simulink model "SkywalkerX8_Longitudinal_Control_Digital"  (R2018a)
settings: Solver=FixedStepAuto  StartTime=0.0  StopTime=inf  FixedStep=0.001  RelTol=1e-3
undefined symbols (not defined in the file): DiscIntNeverNeededParam, SkywalkerX8
libraries: simulink_extras x4
settings Model: EnablePacing=on  Creator=David  LastModifiedBy=David

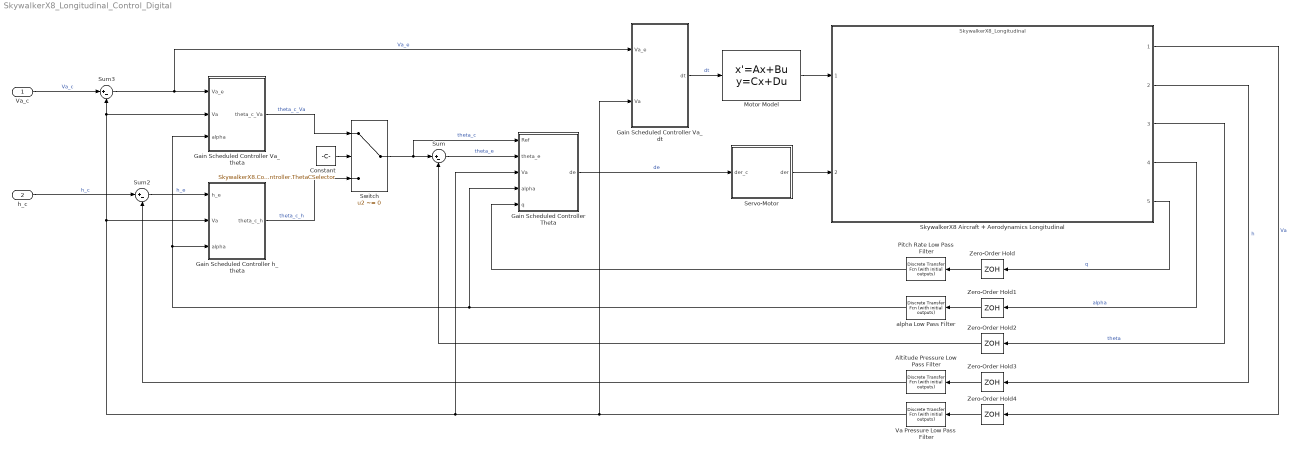
== system SkywalkerX8_Longitudinal_Control_Digital ==
  Va_c : Inport
  h_c : Inport  Port=2
  Altitude Pressure Low Pass Filter : simulink_extras/Additional Discrete/Discrete Transfer Fcn (with initial outputs)  N=cell2mat(SkywalkerX8.Sensors.Filters.AltitudePressure.FilterTFDigital.Numerator)  D=cell2mat(SkywalkerX8.Sensors.Filters.AltitudePressure.FilterTFDigital.Denominator)  U0=-SkywalkerX8.InitialConditions.XeYeZe(3)  Y0=-SkywalkerX8.InitialConditions.XeYeZe(3)  TS=SkywalkerX8.Sensors.Filters.AltitudePressure.FilterSampleTime
      settings: SourceProductName=Simulink  SourceProductBaseCode=SL
  Constant : Constant  Value=SkywalkerX8.Control.Longitudinal.AlgebraicDesign.ReducedOrderModel.Controller.ThetaCSelector
  Gain Scheduled Controller Theta : Subsystem
  Gain Scheduled Controller Va_dt : Subsystem
  Gain Scheduled Controller Va_theta : Subsystem
  Gain Scheduled Controller h_theta : Subsystem
  Motor Model : StateSpace  A=SkywalkerX8.Actuators.Motor.SS.A  B=SkywalkerX8.Actuators.Motor.SS.B  C=SkywalkerX8.Actuators.Motor.SS.C  D=SkywalkerX8.Actuators.Motor.SS.D  InitialCondition=SkywalkerX8.InitialConditions.dt/SkywalkerX8.Actuators.Motor.SS.C
      mask Display: image('motor.jpg', 'center')
  Pitch Rate Low Pass Filter : simulink_extras/Additional Discrete/Discrete Transfer Fcn (with initial outputs)  N=cell2mat(SkywalkerX8.Sensors.Filters.AngularRates.Pitch.FilterTFDigital.Numerator)  D=cell2mat(SkywalkerX8.Sensors.Filters.AngularRates.Pitch.FilterTFDigital.Denominator)  U0=SkywalkerX8.Sensors.Filters.AngularRates.Pitch.InitialCondition  Y0=SkywalkerX8.Sensors.Filters.AngularRates.Pitch.InitialCondition  TS=SkywalkerX8.Sensors.Filters.AngularRates.Pitch.FilterSampleTime
      settings: SourceProductName=Simulink  SourceProductBaseCode=SL
  Servo-Motor : Subsystem
      mask Display: image('servo.jpg', 'center')
  SkywalkerX8 Aircraft + Aerodynamics Longitudinal : ModelReference  ModelNameDialog=SkywalkerX8_Longitudinal  ModelReferenceVersion=1.60
      mask Display:
      | image('x8SkySunset.png', 'center')
      | 
      | port_label('input', 1, '\delta_t (Unitless)', 'texmode', 'on')
      | port_label('input', 2, '\delta_e (rad)', 'texmode', 'on')
      | 
      | port_label('output', 1, 'V_a (m/s)', 'texmode', 'on')
      | port_label('output', 2, 'Altitude (m)', 'texmode', 'on')
      | port_label('output', 3, '\theta (rad)', 'texmode', 'on')
      | port_label('output', 4, 'alpha (rad)', 'texmode', 'on')
      | port_label('output', 5, 'q (rad/s)', 'texmode', 'on')
  Sum : Sum  Inputs=|+-
  Sum2 : Sum  Inputs=|+-
  Sum3 : Sum  Inputs=|+-
  Switch : Switch  Criteria=u2 ~= 0
  Va Pressure Low Pass Filter : simulink_extras/Additional Discrete/Discrete Transfer Fcn (with initial outputs)  N=cell2mat(SkywalkerX8.Sensors.Filters.AirspeedPressure.FilterTFDigital.Numerator)  D=cell2mat(SkywalkerX8.Sensors.Filters.AirspeedPressure.FilterTFDigital.Denominator)  U0=sqrt(SkywalkerX8.InitialConditions.uvw*SkywalkerX8.InitialConditions.uvw')  Y0=sqrt(SkywalkerX8.InitialConditions.uvw*SkywalkerX8.InitialConditions.uvw')  TS=SkywalkerX8.Sensors.Filters.AirspeedPressure.FilterSampleTime
      settings: SourceProductName=Simulink  SourceProductBaseCode=SL
  Zero-Order Hold : ZeroOrderHold  SampleTime=SkywalkerX8.Sensors.IMU.Gyroscope.SampleTime
  Zero-Order Hold1 : ZeroOrderHold  SampleTime=SkywalkerX8.Sensors.AoA.SampleTime
  Zero-Order Hold2 : ZeroOrderHold  SampleTime=SkywalkerX8.Sensors.EKF.GPSSmoothing.StateTransitionSampleTime
  Zero-Order Hold3 : ZeroOrderHold  SampleTime=SkywalkerX8.Sensors.AltitudePressure.SampleTime
  Zero-Order Hold4 : ZeroOrderHold  SampleTime=SkywalkerX8.Sensors.AirspeedPressure.SampleTime
  alpha Low Pass Filter : simulink_extras/Additional Discrete/Discrete Transfer Fcn (with initial outputs)  N=cell2mat(SkywalkerX8.Sensors.Filters.AoA.FilterTFDigital.Numerator)  D=cell2mat(SkywalkerX8.Sensors.Filters.AoA.FilterTFDigital.Denominator)  U0=SkywalkerX8.Sensors.Filters.AoA.InitialCondition  Y0=SkywalkerX8.Sensors.Filters.AoA.InitialCondition  TS=SkywalkerX8.Sensors.Filters.AoA.FilterSampleTime
      settings: SourceProductName=Simulink  SourceProductBaseCode=SL
  wires:
  SkywalkerX8 Aircraft + Aerodynamics Longitudinal/3 -> Zero-Order Hold2/1  "theta"
  SkywalkerX8 Aircraft + Aerodynamics Longitudinal/1 -> Zero-Order Hold4/1  "Va"
  SkywalkerX8 Aircraft + Aerodynamics Longitudinal/2 -> Zero-Order Hold3/1  "h"
  Switch/1 -> Gain Scheduled Controller Theta/1(Ref), Sum/1  "theta_c"
  Va_c/1 -> Sum3/1  "Va_c"
  h_c/1 -> Sum2/1  "h_c"
  Gain Scheduled Controller Va_theta/1(theta_c_Va) -> Switch/1  "theta_c_Va"
  Sum3/1 -> Gain Scheduled Controller Va_theta/1(Va_e), Gain Scheduled Controller Va_dt/1(Va_e)  "Va_e"
  Gain Scheduled Controller h_theta/1(theta_c_h) -> Switch/3  "theta_c_h"
  Sum/1 -> Gain Scheduled Controller Theta/2(theta_e)  "theta_e"
  Sum2/1 -> Gain Scheduled Controller h_theta/1(h_e)  "h_e"
  SkywalkerX8 Aircraft + Aerodynamics Longitudinal/4 -> Zero-Order Hold1/1  "alpha"
  Constant/1 -> Switch/2
  Zero-Order Hold4/1 -> Va Pressure Low Pass Filter/1
  Zero-Order Hold3/1 -> Altitude Pressure Low Pass Filter/1
  Zero-Order Hold2/1 -> Sum/2
  Zero-Order Hold1/1 -> alpha Low Pass Filter/1
  SkywalkerX8 Aircraft + Aerodynamics Longitudinal/5 -> Zero-Order Hold/1  "q"
  Gain Scheduled Controller Theta/1(de) -> Servo-Motor/1(der_c)  "de"
  Zero-Order Hold/1 -> Pitch Rate Low Pass Filter/1
  Gain Scheduled Controller Va_dt/1(dt) -> Motor Model/1  "dt"
  Motor Model/1 -> SkywalkerX8 Aircraft + Aerodynamics Longitudinal/1
  Servo-Motor/1(der) -> SkywalkerX8 Aircraft + Aerodynamics Longitudinal/2
  Pitch Rate Low Pass Filter/1 -> Gain Scheduled Controller Theta/5(q)
  alpha Low Pass Filter/1 -> Gain Scheduled Controller Theta/4(alpha), Gain Scheduled Controller Va_theta/3(alpha), Gain Scheduled Controller h_theta/3(alpha)
  Altitude Pressure Low Pass Filter/1 -> Sum2/2
  Va Pressure Low Pass Filter/1 -> Gain Scheduled Controller Va_dt/2(Va), Gain Scheduled Controller Theta/3(Va), Gain Scheduled Controller h_theta/2(Va), Gain Scheduled Controller Va_theta/2(Va), Sum3/2

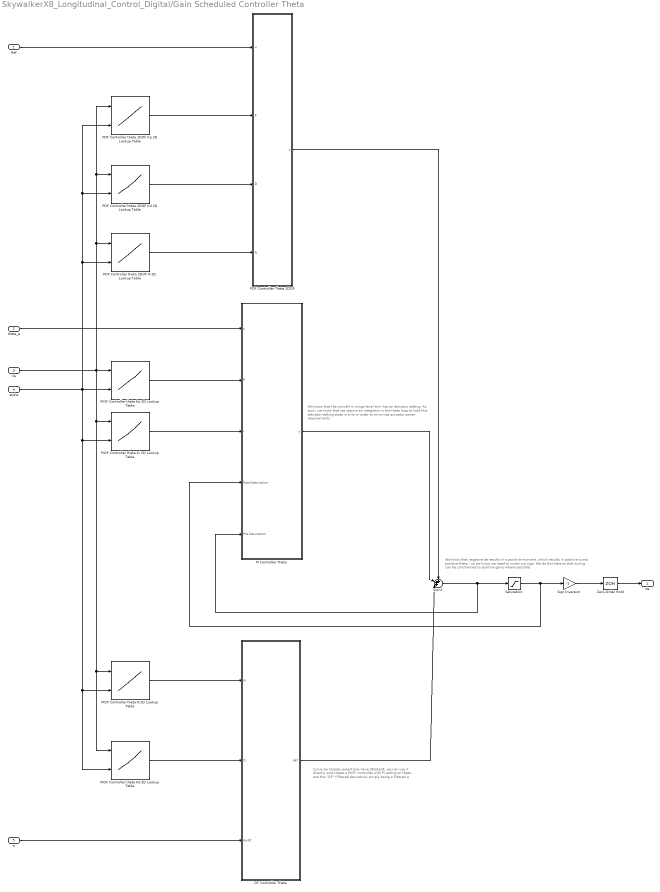
== system SkywalkerX8_Longitudinal_Control_Digital/Gain Scheduled Controller Theta ==
  note: Since we already essentially have dtheta/dt,
      | we can use it directly and create a PIDF controller
      | with PI acting on theta and the "DF" (filtered derivative)
      | simply being a filtered q
  note: We know that negative de results in a positive moment, which results in
      | positive q and positive theta - so we know we need to invert our sign.
      | We do this here so that tuning can be constrained to positive gains where possible.
  note: We know that the aircraft in wings-level trim has an elevator setting. As such, we know that we require an integrator in the theta loop to hold this elevator setting state in trim in order to minimize actuator power requirements.
  Ref : Inport
  theta_e : Inport  Port=2
  Va : Inport  Port=3
  alpha : Inport  Port=4
  q : Inport  Port=5
  DF Controller Theta : Subsystem
  PDF Controller Theta 2DOF : Subsystem
  PDF Controller theta 2DOF Kd 2D Lookup Table : Lookup_n-D  BreakpointsForDimension1=SkywalkerX8.Control.Longitudinal.SchedulingVariables.VaArray  BreakpointsForDimension2=SkywalkerX8.Control.Longitudinal.SchedulingVariables.alphaArray  Table=SkywalkerX8.Control.Longitudinal.thetaController.Digital.KdTheta2DOF  InternalRulePriority=Speed  RndMeth=Simplest  InputSameDT=on
  PDF Controller theta 2DOF Kp 2D Lookup Table : Lookup_n-D  BreakpointsForDimension1=SkywalkerX8.Control.Longitudinal.SchedulingVariables.VaArray  BreakpointsForDimension2=SkywalkerX8.Control.Longitudinal.SchedulingVariables.alphaArray  Table=SkywalkerX8.Control.Longitudinal.thetaController.Digital.KpTheta2DOF  InternalRulePriority=Speed  RndMeth=Simplest  InputSameDT=on
  PDF Controller theta 2DOF N 2D Lookup Table : Lookup_n-D  BreakpointsForDimension1=SkywalkerX8.Control.Longitudinal.SchedulingVariables.VaArray  BreakpointsForDimension2=SkywalkerX8.Control.Longitudinal.SchedulingVariables.alphaArray  Table=SkywalkerX8.Control.Longitudinal.thetaController.Digital.NTheta2DOF  InternalRulePriority=Speed  RndMeth=Simplest  InputSameDT=on
  PI Controller Theta : Subsystem
  PIDF Controller theta Kd 2D Lookup Table : Lookup_n-D  BreakpointsForDimension1=SkywalkerX8.Control.Longitudinal.SchedulingVariables.VaArray  BreakpointsForDimension2=SkywalkerX8.Control.Longitudinal.SchedulingVariables.alphaArray  Table=SkywalkerX8.Control.Longitudinal.thetaController.Digital.KdTheta  InternalRulePriority=Speed  RndMeth=Simplest  InputSameDT=on
  PIDF Controller theta Ki 2D Lookup Table : Lookup_n-D  BreakpointsForDimension1=SkywalkerX8.Control.Longitudinal.SchedulingVariables.VaArray  BreakpointsForDimension2=SkywalkerX8.Control.Longitudinal.SchedulingVariables.alphaArray  Table=SkywalkerX8.Control.Longitudinal.thetaController.Digital.KiTheta  InternalRulePriority=Speed  RndMeth=Simplest  InputSameDT=on
  PIDF Controller theta Kp 2D Lookup Table : Lookup_n-D  BreakpointsForDimension1=SkywalkerX8.Control.Longitudinal.SchedulingVariables.VaArray  BreakpointsForDimension2=SkywalkerX8.Control.Longitudinal.SchedulingVariables.alphaArray  Table=SkywalkerX8.Control.Longitudinal.thetaController.Digital.KpTheta  InternalRulePriority=Speed  RndMeth=Simplest  InputSameDT=on
  PIDF Controller theta N 2D Lookup Table : Lookup_n-D  BreakpointsForDimension1=SkywalkerX8.Control.Longitudinal.SchedulingVariables.VaArray  BreakpointsForDimension2=SkywalkerX8.Control.Longitudinal.SchedulingVariables.alphaArray  Table=SkywalkerX8.Control.Longitudinal.thetaController.Digital.NTheta  InternalRulePriority=Speed  RndMeth=Simplest  InputSameDT=on
  Saturation : Saturate  UpperLimit=SkywalkerX8.Control.Longitudinal.thetaController.Digital.upperSaturationNegativeDe  LowerLimit=SkywalkerX8.Control.Longitudinal.thetaController.Digital.lowerSaturationNegativeDe
  Sign Inversion : Gain  Gain=-1
  Sum1 : Sum  Inputs=+++|
  Zero-Order Hold : ZeroOrderHold  SampleTime=SkywalkerX8.Control.Longitudinal.thetaController.Digital.SampleTime
  de : Outport
  wires:
  Va/1 -> PDF Controller theta 2DOF Kd 2D Lookup Table/1, PDF Controller theta 2DOF Kp 2D Lookup Table/1, PDF Controller theta 2DOF N 2D Lookup Table/1, PIDF Controller theta N 2D Lookup Table/1, PIDF Controller theta Kd 2D Lookup Table/1, PIDF Controller theta Ki 2D Lookup Table/1, PIDF Controller theta Kp 2D Lookup Table/1
  theta_e/1 -> PI Controller Theta/1(u)
  PIDF Controller theta Kp 2D Lookup Table/1 -> PI Controller Theta/2(P)
  PIDF Controller theta Ki 2D Lookup Table/1 -> PI Controller Theta/3(I)
  alpha/1 -> PDF Controller theta 2DOF N 2D Lookup Table/2, PDF Controller theta 2DOF Kd 2D Lookup Table/2, PDF Controller theta 2DOF Kp 2D Lookup Table/2, PIDF Controller theta N 2D Lookup Table/2, PIDF Controller theta Kd 2D Lookup Table/2, PIDF Controller theta Ki 2D Lookup Table/2, PIDF Controller theta Kp 2D Lookup Table/2
  PI Controller Theta/1(y) -> Sum1/2
  Sum1/1 -> Saturation/1, PI Controller Theta/5(Pre-Saturation)
  Saturation/1 -> Sign Inversion/1, PI Controller Theta/4(Post-Saturation)
  PIDF Controller theta N 2D Lookup Table/1 -> DF Controller Theta/1(N)
  PIDF Controller theta Kd 2D Lookup Table/1 -> DF Controller Theta/2(D)
  q/1 -> DF Controller Theta/3(du/dt)
  DF Controller Theta/1(de*) -> Sum1/3
  Sign Inversion/1 -> Zero-Order Hold/1
  PDF Controller theta 2DOF Kp 2D Lookup Table/1 -> PDF Controller Theta 2DOF/2(P)
  PDF Controller theta 2DOF Kd 2D Lookup Table/1 -> PDF Controller Theta 2DOF/3(D)
  PDF Controller theta 2DOF N 2D Lookup Table/1 -> PDF Controller Theta 2DOF/4(N)
  Ref/1 -> PDF Controller Theta 2DOF/1(u)
  PDF Controller Theta 2DOF/1(y) -> Sum1/1
  Zero-Order Hold/1 -> de/1

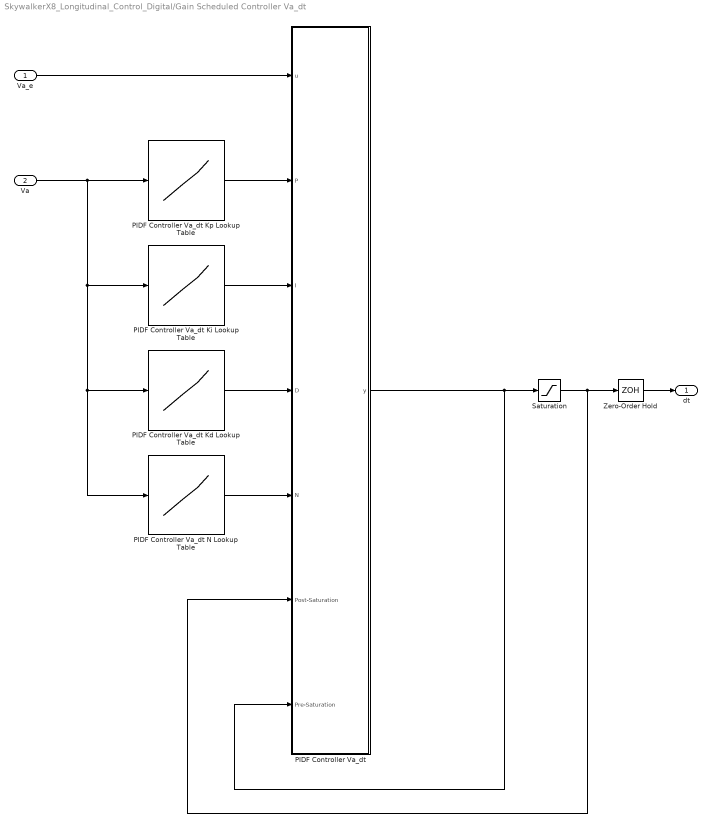
== system SkywalkerX8_Longitudinal_Control_Digital/Gain Scheduled Controller Va_dt ==
  Va_e : Inport
  Va : Inport  Port=2
  PIDF Controller Va_dt : Subsystem
  PIDF Controller Va_dt Kd Lookup Table : Lookup_n-D  NumberOfTableDimensions=1  BreakpointsForDimension1=SkywalkerX8.Control.Longitudinal.SchedulingVariables.VaArray  BreakpointsForDimension2=[1 2 3 4 5]  Table=SkywalkerX8.Control.Longitudinal.VaDtController.Digital.KdVaDt  InternalRulePriority=Speed  RndMeth=Simplest  InputSameDT=on
  PIDF Controller Va_dt Ki Lookup Table : Lookup_n-D  NumberOfTableDimensions=1  BreakpointsForDimension1=SkywalkerX8.Control.Longitudinal.SchedulingVariables.VaArray  BreakpointsForDimension2=[1 2 3 4 5]  Table=SkywalkerX8.Control.Longitudinal.VaDtController.Digital.KiVaDt  InternalRulePriority=Speed  RndMeth=Simplest  InputSameDT=on
  PIDF Controller Va_dt Kp Lookup Table : Lookup_n-D  NumberOfTableDimensions=1  BreakpointsForDimension1=SkywalkerX8.Control.Longitudinal.SchedulingVariables.VaArray  BreakpointsForDimension2=[1 2 3 4 5]  Table=SkywalkerX8.Control.Longitudinal.VaDtController.Digital.KpVaDt  InternalRulePriority=Speed  RndMeth=Simplest  InputSameDT=on
  PIDF Controller Va_dt N Lookup Table : Lookup_n-D  NumberOfTableDimensions=1  BreakpointsForDimension1=SkywalkerX8.Control.Longitudinal.SchedulingVariables.VaArray  BreakpointsForDimension2=[1 2 3 4 5]  Table=SkywalkerX8.Control.Longitudinal.VaDtController.Digital.NVaDt  InternalRulePriority=Speed  RndMeth=Simplest  InputSameDT=on
  Saturation : Saturate  UpperLimit=SkywalkerX8.Control.Longitudinal.VaDtController.upperSaturationDt  LowerLimit=SkywalkerX8.Control.Longitudinal.VaDtController.lowerSaturationDt
  Zero-Order Hold : ZeroOrderHold  SampleTime=SkywalkerX8.Control.Longitudinal.VaDtController.Digital.SampleTime
  dt : Outport
  wires:
  Va_e/1 -> PIDF Controller Va_dt/1(u)
  Saturation/1 -> PIDF Controller Va_dt/6(Post-Saturation), Zero-Order Hold/1
  PIDF Controller Va_dt Kp Lookup Table/1 -> PIDF Controller Va_dt/2(P)
  Va/1 -> PIDF Controller Va_dt Kp Lookup Table/1, PIDF Controller Va_dt N Lookup Table/1, PIDF Controller Va_dt Kd Lookup Table/1, PIDF Controller Va_dt Ki Lookup Table/1
  PIDF Controller Va_dt Ki Lookup Table/1 -> PIDF Controller Va_dt/3(I)
  PIDF Controller Va_dt Kd Lookup Table/1 -> PIDF Controller Va_dt/4(D)
  PIDF Controller Va_dt N Lookup Table/1 -> PIDF Controller Va_dt/5(N)
  PIDF Controller Va_dt/1(y) -> Saturation/1, PIDF Controller Va_dt/7(Pre-Saturation)
  Zero-Order Hold/1 -> dt/1

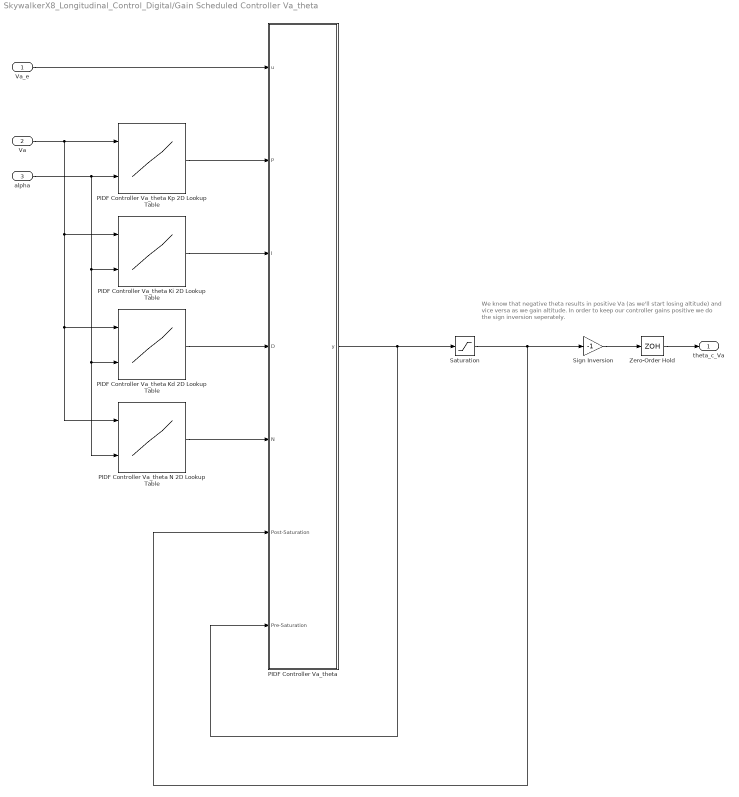
== system SkywalkerX8_Longitudinal_Control_Digital/Gain Scheduled Controller Va_theta ==
  note: We know that negative theta results in positive Va (as we'll start losing altitude)
      | and vice versa as we gain altitude. In order to keep our controller gains positive
      |  we do the sign inversion seperately.
  Va_e : Inport
  Va : Inport  Port=2
  alpha : Inport  Port=3
  PIDF Controller Va_theta : Subsystem
  PIDF Controller Va_theta Kd 2D Lookup Table : Lookup_n-D  BreakpointsForDimension1=SkywalkerX8.Control.Longitudinal.SchedulingVariables.VaArray  BreakpointsForDimension2=SkywalkerX8.Control.Longitudinal.SchedulingVariables.alphaArray  Table=SkywalkerX8.Control.Longitudinal.VaThetaController.Digital.KdVaTheta  InternalRulePriority=Speed  RndMeth=Simplest  InputSameDT=on
  PIDF Controller Va_theta Ki 2D Lookup Table : Lookup_n-D  BreakpointsForDimension1=SkywalkerX8.Control.Longitudinal.SchedulingVariables.VaArray  BreakpointsForDimension2=SkywalkerX8.Control.Longitudinal.SchedulingVariables.alphaArray  Table=SkywalkerX8.Control.Longitudinal.VaThetaController.Digital.KiVaTheta  InternalRulePriority=Speed  RndMeth=Simplest  InputSameDT=on
  PIDF Controller Va_theta Kp 2D Lookup Table : Lookup_n-D  BreakpointsForDimension1=SkywalkerX8.Control.Longitudinal.SchedulingVariables.VaArray  BreakpointsForDimension2=SkywalkerX8.Control.Longitudinal.SchedulingVariables.alphaArray  Table=SkywalkerX8.Control.Longitudinal.VaThetaController.Digital.KpVaTheta  InternalRulePriority=Speed  RndMeth=Simplest  InputSameDT=on
  PIDF Controller Va_theta N 2D Lookup Table : Lookup_n-D  BreakpointsForDimension1=SkywalkerX8.Control.Longitudinal.SchedulingVariables.VaArray  BreakpointsForDimension2=SkywalkerX8.Control.Longitudinal.SchedulingVariables.alphaArray  Table=SkywalkerX8.Control.Longitudinal.VaThetaController.Digital.NVaTheta  InternalRulePriority=Speed  RndMeth=Simplest  InputSameDT=on
  Saturation : Saturate  UpperLimit=SkywalkerX8.Control.Longitudinal.VaThetaController.Digital.upperSaturationThetaC  LowerLimit=SkywalkerX8.Control.Longitudinal.VaThetaController.Digital.lowerSaturationThetaC
  Sign Inversion : Gain  Gain=-1
  Zero-Order Hold : ZeroOrderHold  SampleTime=SkywalkerX8.Control.Longitudinal.altController.Digital.SampleTime
  theta_c_Va : Outport
  wires:
  Va_e/1 -> PIDF Controller Va_theta/1(u)
  Saturation/1 -> Sign Inversion/1, PIDF Controller Va_theta/6(Post-Saturation)
  PIDF Controller Va_theta Kp 2D Lookup Table/1 -> PIDF Controller Va_theta/2(P)
  Va/1 -> PIDF Controller Va_theta Kd 2D Lookup Table/1, PIDF Controller Va_theta N 2D Lookup Table/1, PIDF Controller Va_theta Ki 2D Lookup Table/1, PIDF Controller Va_theta Kp 2D Lookup Table/1
  PIDF Controller Va_theta Ki 2D Lookup Table/1 -> PIDF Controller Va_theta/3(I)
  PIDF Controller Va_theta Kd 2D Lookup Table/1 -> PIDF Controller Va_theta/4(D)
  PIDF Controller Va_theta N 2D Lookup Table/1 -> PIDF Controller Va_theta/5(N)
  alpha/1 -> PIDF Controller Va_theta N 2D Lookup Table/2, PIDF Controller Va_theta Kd 2D Lookup Table/2, PIDF Controller Va_theta Ki 2D Lookup Table/2, PIDF Controller Va_theta Kp 2D Lookup Table/2
  Sign Inversion/1 -> Zero-Order Hold/1
  PIDF Controller Va_theta/1(y) -> Saturation/1, PIDF Controller Va_theta/7(Pre-Saturation)
  Zero-Order Hold/1 -> theta_c_Va/1

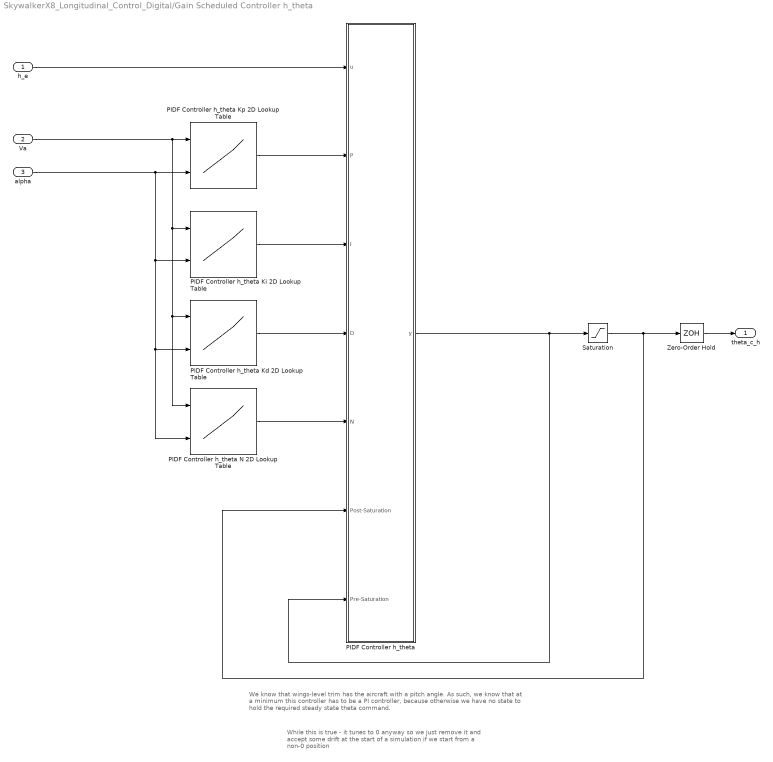
== system SkywalkerX8_Longitudinal_Control_Digital/Gain Scheduled Controller h_theta ==
  note: While this is true - it tunes to 0 anyway so we just remove it
      | and accept some drift at the start of a simulation if we start
      | from a non-0 position
  note: We know that wings-level trim has the aircraft with a pitch angle. As such,
      | we know that at a minimum this controller has to be a PI controller, because otherwise
      | we have no state to hold the required steady state theta command.
  h_e : Inport
  Va : Inport  Port=2
  alpha : Inport  Port=3
  PIDF Controller h_theta : Subsystem
  PIDF Controller h_theta Kd 2D Lookup Table : Lookup_n-D  BreakpointsForDimension1=SkywalkerX8.Control.Longitudinal.SchedulingVariables.VaArray  BreakpointsForDimension2=SkywalkerX8.Control.Longitudinal.SchedulingVariables.alphaArray  Table=SkywalkerX8.Control.Longitudinal.altController.Digital.KdAlt  InternalRulePriority=Speed  RndMeth=Simplest  InputSameDT=on
  PIDF Controller h_theta Ki 2D Lookup Table : Lookup_n-D  BreakpointsForDimension1=SkywalkerX8.Control.Longitudinal.SchedulingVariables.VaArray  BreakpointsForDimension2=SkywalkerX8.Control.Longitudinal.SchedulingVariables.alphaArray  Table=SkywalkerX8.Control.Longitudinal.altController.Digital.KiAlt  InternalRulePriority=Speed  RndMeth=Simplest  InputSameDT=on
  PIDF Controller h_theta Kp 2D Lookup Table : Lookup_n-D  BreakpointsForDimension1=SkywalkerX8.Control.Longitudinal.SchedulingVariables.VaArray  BreakpointsForDimension2=SkywalkerX8.Control.Longitudinal.SchedulingVariables.alphaArray  Table=SkywalkerX8.Control.Longitudinal.altController.Digital.KpAlt  InternalRulePriority=Speed  RndMeth=Simplest  InputSameDT=on
  PIDF Controller h_theta N 2D Lookup Table : Lookup_n-D  BreakpointsForDimension1=SkywalkerX8.Control.Longitudinal.SchedulingVariables.VaArray  BreakpointsForDimension2=SkywalkerX8.Control.Longitudinal.SchedulingVariables.alphaArray  Table=SkywalkerX8.Control.Longitudinal.altController.Digital.NAlt  InternalRulePriority=Speed  RndMeth=Simplest  InputSameDT=on
  Saturation : Saturate  UpperLimit=SkywalkerX8.Control.Longitudinal.altController.Digital.upperSaturationThetaC  LowerLimit=SkywalkerX8.Control.Longitudinal.altController.Digital.lowerSaturationThetaC
  Zero-Order Hold : ZeroOrderHold  SampleTime=SkywalkerX8.Control.Longitudinal.altController.Digital.SampleTime
  theta_c_h : Outport
  wires:
  PIDF Controller h_theta Kp 2D Lookup Table/1 -> PIDF Controller h_theta/2(P)
  alpha/1 -> PIDF Controller h_theta N 2D Lookup Table/2, PIDF Controller h_theta Kd 2D Lookup Table/2, PIDF Controller h_theta Ki 2D Lookup Table/2, PIDF Controller h_theta Kp 2D Lookup Table/2
  h_e/1 -> PIDF Controller h_theta/1(u)
  Va/1 -> PIDF Controller h_theta N 2D Lookup Table/1, PIDF Controller h_theta Kd 2D Lookup Table/1, PIDF Controller h_theta Ki 2D Lookup Table/1, PIDF Controller h_theta Kp 2D Lookup Table/1
  PIDF Controller h_theta Kd 2D Lookup Table/1 -> PIDF Controller h_theta/4(D)
  PIDF Controller h_theta N 2D Lookup Table/1 -> PIDF Controller h_theta/5(N)
  Saturation/1 -> PIDF Controller h_theta/6(Post-Saturation), Zero-Order Hold/1
  PIDF Controller h_theta/1(y) -> PIDF Controller h_theta/7(Pre-Saturation), Saturation/1
  PIDF Controller h_theta Ki 2D Lookup Table/1 -> PIDF Controller h_theta/3(I)
  Zero-Order Hold/1 -> theta_c_h/1

== system SkywalkerX8_Longitudinal_Control_Digital/Servo-Motor ==
  der_c : Inport
  Rate Limiter : RateLimiter  RisingSlewLimit=SkywalkerX8.Actuators.Servos.RateLimit  FallingSlewLimit=-SkywalkerX8.Actuators.Servos.RateLimit  InitialCondition=SkywalkerX8.InitialConditions.de
  Second Order Servo-Motor Model : StateSpace  A=SkywalkerX8.Actuators.Servos.SS.A  B=SkywalkerX8.Actuators.Servos.SS.B  C=SkywalkerX8.Actuators.Servos.SS.C  D=SkywalkerX8.Actuators.Servos.SS.D  InitialCondition=SkywalkerX8.InitialConditions.de/SkywalkerX8.Actuators.Servos.SS.C(2)
  der : Outport
  wires:
  der_c/1 -> Second Order Servo-Motor Model/1
  Second Order Servo-Motor Model/1 -> Rate Limiter/1
  Rate Limiter/1 -> der/1

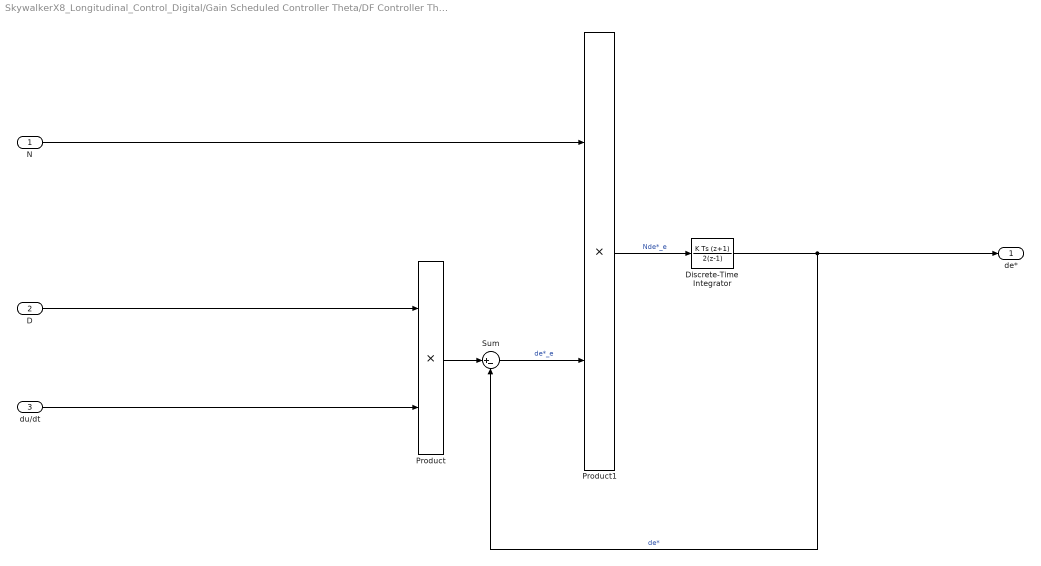
== system SkywalkerX8_Longitudinal_Control_Digital/Gain Scheduled Controller Theta/DF Controller Theta ==
  N : Inport
  D : Inport  Port=2
  du/dt : Inport  Port=3
  Discrete-Time Integrator : DiscreteIntegrator  IntegratorMethod=Integration: Trapezoidal  SampleTime=SkywalkerX8.Control.Longitudinal.thetaController.Digital.SampleTime  ICPrevOutput=DiscIntNeverNeededParam  ICPrevScaledInput=DiscIntNeverNeededParam
  Product : Product
  Product1 : Product
  Sum : Sum  Inputs=|+-
  de* : Outport
  wires:
  Discrete-Time Integrator/1 -> de*/1, Sum/2  "de*"
  Product1/1 -> Discrete-Time Integrator/1  "Nde*_e"
  du/dt/1 -> Product/2
  D/1 -> Product/1
  Sum/1 -> Product1/2  "de*_e"
  N/1 -> Product1/1
  Product/1 -> Sum/1

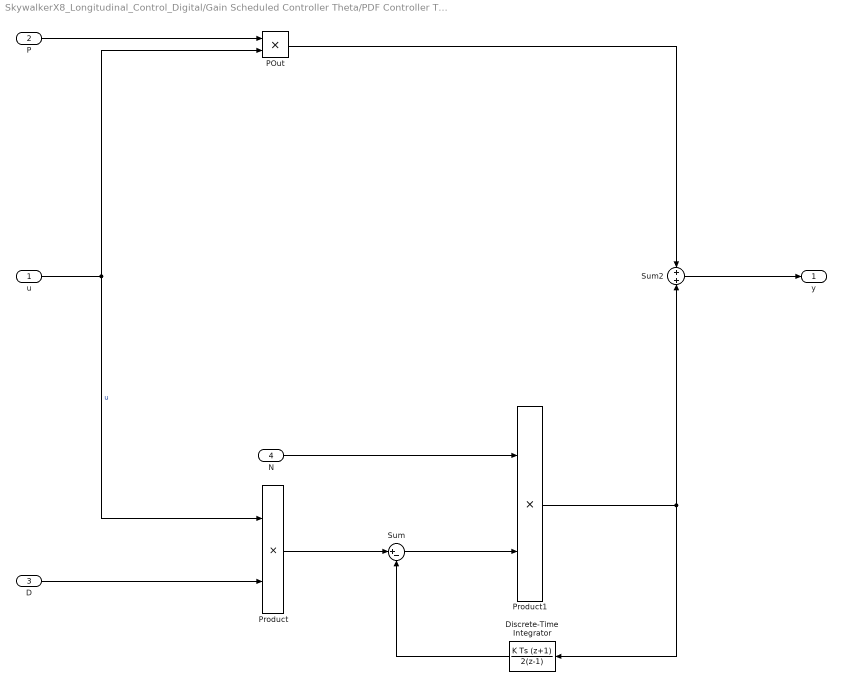
== system SkywalkerX8_Longitudinal_Control_Digital/Gain Scheduled Controller Theta/PDF Controller Theta 2DOF ==
  u : Inport
  P : Inport  Port=2
  D : Inport  Port=3
  N : Inport  Port=4
  Discrete-Time Integrator : DiscreteIntegrator  IntegratorMethod=Integration: Trapezoidal  SampleTime=SkywalkerX8.Control.Longitudinal.thetaController.Digital.SampleTime  ICPrevOutput=DiscIntNeverNeededParam  ICPrevScaledInput=DiscIntNeverNeededParam
  POut : Product
  Product : Product
  Product1 : Product
  Sum : Sum  Inputs=|+-
  Sum2 : Sum
  y : Outport  InitialOutput=0
  wires:
  Sum2/1 -> y/1
  N/1 -> Product1/1
  Product1/1 -> Discrete-Time Integrator/1, Sum2/2
  Sum/1 -> Product1/2
  POut/1 -> Sum2/1
  D/1 -> Product/2
  u/1 -> Product/1, POut/2  "u"
  Discrete-Time Integrator/1 -> Sum/2
  Product/1 -> Sum/1
  P/1 -> POut/1

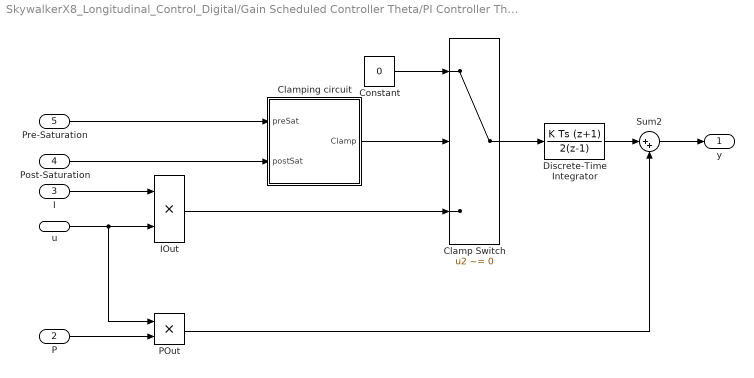
== system SkywalkerX8_Longitudinal_Control_Digital/Gain Scheduled Controller Theta/PI Controller Theta ==
  u : Inport
  P : Inport  Port=2
  I : Inport  Port=3
  Post-Saturation : Inport  Port=4
  Pre-Saturation : Inport  Port=5
  Clamp Switch : Switch  Criteria=u2 ~= 0
  Clamping circuit : Subsystem
  Constant : Constant  Value=0
  Discrete-Time Integrator : DiscreteIntegrator  IntegratorMethod=Integration: Trapezoidal  InitialCondition=SkywalkerX8.InitialConditions.ThetaController.Integrator  SampleTime=SkywalkerX8.Control.Longitudinal.thetaController.Digital.SampleTime  ICPrevOutput=DiscIntNeverNeededParam  ICPrevScaledInput=DiscIntNeverNeededParam
  IOut : Product  DisableCoverage=on
  POut : Product
  Sum2 : Sum  Inputs=|++
  y : Outport  InitialOutput=0
  wires:
  IOut/1 -> Clamp Switch/3
  Clamp Switch/1 -> Discrete-Time Integrator/1
  Sum2/1 -> y/1
  Pre-Saturation/1 -> Clamping circuit/1(preSat)
  Post-Saturation/1 -> Clamping circuit/2(postSat)
  Clamping circuit/1(Clamp) -> Clamp Switch/2
  Constant/1 -> Clamp Switch/1
  Discrete-Time Integrator/1 -> Sum2/1
  POut/1 -> Sum2/2
  P/1 -> POut/2
  u/1 -> POut/1, IOut/2
  I/1 -> IOut/1

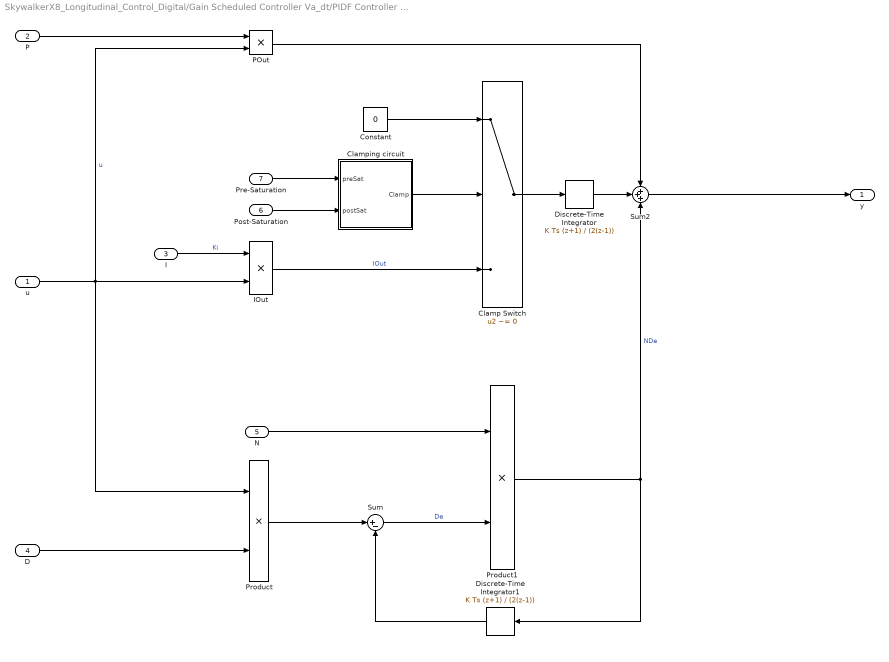
== system SkywalkerX8_Longitudinal_Control_Digital/Gain Scheduled Controller Va_dt/PIDF Controller Va_dt ==
  u : Inport
  P : Inport  Port=2
  I : Inport  Port=3
  D : Inport  Port=4
  N : Inport  Port=5
  Post-Saturation : Inport  Port=6
  Pre-Saturation : Inport  Port=7
  Clamp Switch : Switch  Criteria=u2 ~= 0
  Clamping circuit : Subsystem
  Constant : Constant  Value=0
  Discrete-Time Integrator : DiscreteIntegrator  IntegratorMethod=Integration: Trapezoidal  InitialCondition=SkywalkerX8.InitialConditions.dt  SampleTime=SkywalkerX8.Control.Longitudinal.VaDtController.Digital.SampleTime  ICPrevOutput=DiscIntNeverNeededParam  ICPrevScaledInput=DiscIntNeverNeededParam
  Discrete-Time Integrator1 : DiscreteIntegrator  IntegratorMethod=Integration: Trapezoidal  SampleTime=SkywalkerX8.Control.Longitudinal.VaDtController.Digital.SampleTime  ICPrevOutput=DiscIntNeverNeededParam  ICPrevScaledInput=DiscIntNeverNeededParam
  IOut : Product  DisableCoverage=on
  POut : Product
  Product : Product
  Product1 : Product
  Sum : Sum  Inputs=|+-
  Sum2 : Sum  Inputs=+++
  y : Outport  InitialOutput=0
  wires:
  Sum2/1 -> y/1
  N/1 -> Product1/1
  Product1/1 -> Sum2/3, Discrete-Time Integrator1/1  "NDe"
  Sum/1 -> Product1/2  "De"
  POut/1 -> Sum2/1
  D/1 -> Product/2
  u/1 -> POut/2, Product/1, IOut/2  "u"
  Discrete-Time Integrator1/1 -> Sum/2
  Clamp Switch/1 -> Discrete-Time Integrator/1
  Product/1 -> Sum/1
  Discrete-Time Integrator/1 -> Sum2/2
  Constant/1 -> Clamp Switch/1
  I/1 -> IOut/1  "Ki"
  IOut/1 -> Clamp Switch/3  "IOut"
  Clamping circuit/1(Clamp) -> Clamp Switch/2
  P/1 -> POut/1
  Pre-Saturation/1 -> Clamping circuit/1(preSat)
  Post-Saturation/1 -> Clamping circuit/2(postSat)

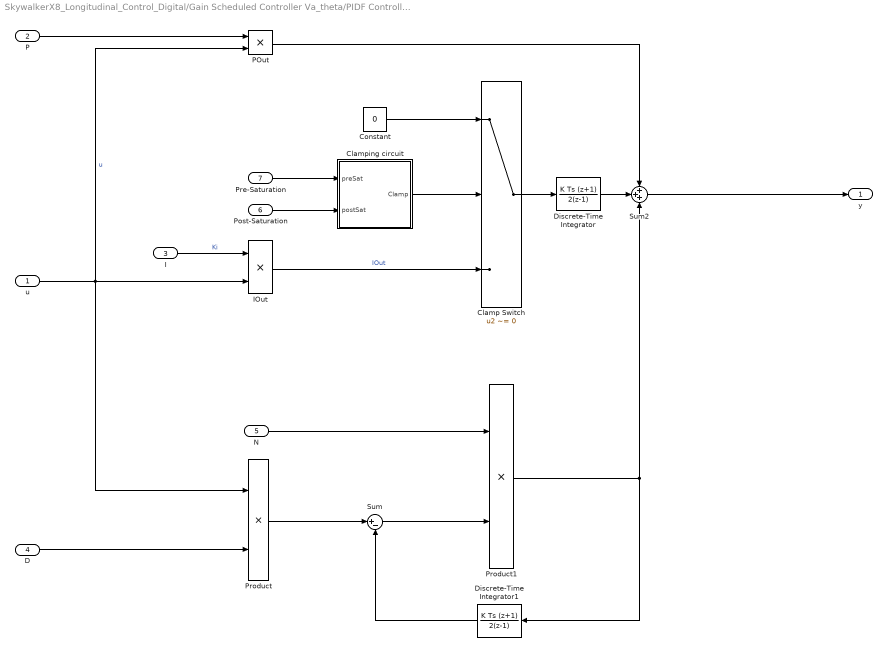
== system SkywalkerX8_Longitudinal_Control_Digital/Gain Scheduled Controller Va_theta/PIDF Controller Va_theta ==
  u : Inport
  P : Inport  Port=2
  I : Inport  Port=3
  D : Inport  Port=4
  N : Inport  Port=5
  Post-Saturation : Inport  Port=6
  Pre-Saturation : Inport  Port=7
  Clamp Switch : Switch  Criteria=u2 ~= 0
  Clamping circuit : Subsystem
  Constant : Constant  Value=0
  Discrete-Time Integrator : DiscreteIntegrator  IntegratorMethod=Integration: Trapezoidal  InitialCondition=-SkywalkerX8.InitialConditions.PhiThetaPsi(2)  SampleTime=SkywalkerX8.Control.Longitudinal.VaThetaController.Digital.SampleTime  ICPrevOutput=DiscIntNeverNeededParam  ICPrevScaledInput=DiscIntNeverNeededParam
  Discrete-Time Integrator1 : DiscreteIntegrator  IntegratorMethod=Integration: Trapezoidal  SampleTime=SkywalkerX8.Control.Longitudinal.VaThetaController.Digital.SampleTime  ICPrevOutput=DiscIntNeverNeededParam  ICPrevScaledInput=DiscIntNeverNeededParam
  IOut : Product  DisableCoverage=on
  POut : Product
  Product : Product
  Product1 : Product
  Sum : Sum  Inputs=|+-
  Sum2 : Sum  Inputs=+++
  y : Outport  InitialOutput=0
  wires:
  Sum2/1 -> y/1
  N/1 -> Product1/1
  Product1/1 -> Discrete-Time Integrator1/1, Sum2/3
  Sum/1 -> Product1/2
  POut/1 -> Sum2/1
  D/1 -> Product/2
  u/1 -> POut/2, Product/1, IOut/2  "u"
  Discrete-Time Integrator1/1 -> Sum/2
  Clamp Switch/1 -> Discrete-Time Integrator/1
  Product/1 -> Sum/1
  Discrete-Time Integrator/1 -> Sum2/2
  Constant/1 -> Clamp Switch/1
  I/1 -> IOut/1  "Ki"
  IOut/1 -> Clamp Switch/3  "IOut"
  Clamping circuit/1(Clamp) -> Clamp Switch/2
  P/1 -> POut/1
  Pre-Saturation/1 -> Clamping circuit/1(preSat)
  Post-Saturation/1 -> Clamping circuit/2(postSat)

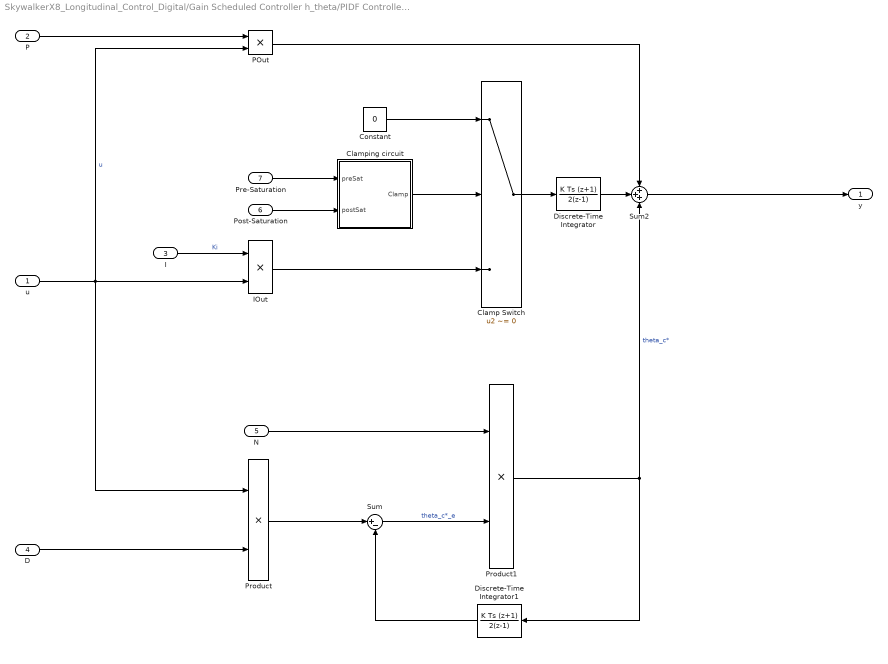
== system SkywalkerX8_Longitudinal_Control_Digital/Gain Scheduled Controller h_theta/PIDF Controller h_theta ==
  u : Inport
  P : Inport  Port=2
  I : Inport  Port=3
  D : Inport  Port=4
  N : Inport  Port=5
  Post-Saturation : Inport  Port=6
  Pre-Saturation : Inport  Port=7
  Clamp Switch : Switch  Criteria=u2 ~= 0
  Clamping circuit : Subsystem
  Constant : Constant  Value=0
  Discrete-Time Integrator : DiscreteIntegrator  IntegratorMethod=Integration: Trapezoidal  InitialCondition=SkywalkerX8.InitialConditions.PhiThetaPsi(2)  SampleTime=SkywalkerX8.Control.Longitudinal.altController.Digital.SampleTime  ICPrevOutput=DiscIntNeverNeededParam  ICPrevScaledInput=DiscIntNeverNeededParam
  Discrete-Time Integrator1 : DiscreteIntegrator  IntegratorMethod=Integration: Trapezoidal  SampleTime=SkywalkerX8.Control.Longitudinal.altController.Digital.SampleTime  ICPrevOutput=DiscIntNeverNeededParam  ICPrevScaledInput=DiscIntNeverNeededParam
  IOut : Product  DisableCoverage=on
  POut : Product
  Product : Product
  Product1 : Product
  Sum : Sum  Inputs=|+-
  Sum2 : Sum  Inputs=+++
  y : Outport  InitialOutput=0
  wires:
  Sum2/1 -> y/1
  N/1 -> Product1/1
  Product1/1 -> Sum2/3, Discrete-Time Integrator1/1  "theta_c*"
  Sum/1 -> Product1/2  "theta_c*_e"
  POut/1 -> Sum2/1
  D/1 -> Product/2
  u/1 -> POut/2, Product/1, IOut/2  "u"
  Discrete-Time Integrator1/1 -> Sum/2
  Clamp Switch/1 -> Discrete-Time Integrator/1
  Product/1 -> Sum/1
  Discrete-Time Integrator/1 -> Sum2/2
  Constant/1 -> Clamp Switch/1
  I/1 -> IOut/1  "Ki"
  IOut/1 -> Clamp Switch/3
  Clamping circuit/1(Clamp) -> Clamp Switch/2
  P/1 -> POut/1
  Pre-Saturation/1 -> Clamping circuit/1(preSat)
  Post-Saturation/1 -> Clamping circuit/2(postSat)

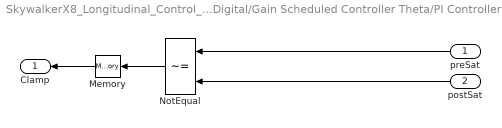
== system SkywalkerX8_Longitudinal_Control_Digital/Gain Scheduled Controller Theta/PI Controller Theta/Clamping circuit ==
  preSat : Inport  DisableCoverage=on
  postSat : Inport  DisableCoverage=on  Port=2
  Memory : Memory  DisableCoverage=on
  NotEqual : RelationalOperator  DisableCoverage=on  Operator=~=  RndMeth=Nearest  InputSameDT=on
  Clamp : Outport  DisableCoverage=on
  wires:
  postSat/1 -> NotEqual/2
  preSat/1 -> NotEqual/1
  NotEqual/1 -> Memory/1
  Memory/1 -> Clamp/1

== system SkywalkerX8_Longitudinal_Control_Digital/Gain Scheduled Controller Va_dt/PIDF Controller Va_dt/Clamping circuit ==
  preSat : Inport  DisableCoverage=on
  postSat : Inport  DisableCoverage=on  Port=2
  Memory : Memory  DisableCoverage=on
  NotEqual : RelationalOperator  DisableCoverage=on  Operator=~=  RndMeth=Nearest  InputSameDT=on
  Clamp : Outport  DisableCoverage=on
  wires:
  postSat/1 -> NotEqual/2
  preSat/1 -> NotEqual/1
  NotEqual/1 -> Memory/1
  Memory/1 -> Clamp/1

== system SkywalkerX8_Longitudinal_Control_Digital/Gain Scheduled Controller Va_theta/PIDF Controller Va_theta/Clamping circuit ==
  preSat : Inport  DisableCoverage=on
  postSat : Inport  DisableCoverage=on  Port=2
  Memory : Memory  DisableCoverage=on
  NotEqual : RelationalOperator  DisableCoverage=on  Operator=~=  RndMeth=Nearest  InputSameDT=on
  Clamp : Outport  DisableCoverage=on
  wires:
  postSat/1 -> NotEqual/2
  preSat/1 -> NotEqual/1
  NotEqual/1 -> Memory/1
  Memory/1 -> Clamp/1

== system SkywalkerX8_Longitudinal_Control_Digital/Gain Scheduled Controller h_theta/PIDF Controller h_theta/Clamping circuit ==
  preSat : Inport  DisableCoverage=on
  postSat : Inport  DisableCoverage=on  Port=2
  Memory : Memory  DisableCoverage=on
  NotEqual : RelationalOperator  DisableCoverage=on  Operator=~=  RndMeth=Nearest  InputSameDT=on
  Clamp : Outport  DisableCoverage=on
  wires:
  postSat/1 -> NotEqual/2
  preSat/1 -> NotEqual/1
  NotEqual/1 -> Memory/1
  Memory/1 -> Clamp/1
